simulink model "Fans_trq"  (R2016b)
settings: configuration reference "CodeGenConfigSet" (kept outside this file)
values from neighbouring files (symbols this model uses):
  Fan_facTrqDemFlt2PT1_C = Calibration.Parameter    [init_Fans_trq.m]    (also in init_Fans_trq_SIL.m = Simulink.Parameter)
  Fan_facTrqDemFltPT1_C = Calibration.Parameter    [init_Fans_trq.m]    (also in init_Fans_trq_SIL.m = Simulink.Parameter)
  Fan_numFans_C = Calibration.Parameter    [init_Fans_trq.m]    (also in init_Fans_trq_SIL.m = Simulink.Parameter)
  Fan_trqDem2_CUR = Calibration.Parameter    [init_Fans_trq.m]    (also in init_Fans_trq_SIL.m = Simulink.Parameter)
  Fan_trqDem2_CURX = Calibration.Parameter    [init_Fans_trq.m]    (also in init_Fans_trq_SIL.m = Simulink.Parameter)
  Fan_trqDem_CUR = Calibration.Parameter    [init_Fans_trq.m]    (also in init_Fans_trq_SIL.m = Simulink.Parameter)
  Fan_trqDem_CURX = Calibration.Parameter    [init_Fans_trq.m]    (also in init_Fans_trq_SIL.m = Simulink.Parameter)
  Fan_trqSplyDem2_C = Calibration.Parameter    [init_Fans_trq.m]    (also in init_Fans_trq_SIL.m = Simulink.Parameter)
  Fan_trqSplyDem_C = Calibration.Parameter    [init_Fans_trq.m]    (also in init_Fans_trq_SIL.m = Simulink.Parameter)
undefined symbols (not defined in the file or in its folder): FanCtl_facCorSpd_MAP_CURX
libraries: CXLib x4
settings Model: Creator=xinchangran  LastModifiedBy=xinchangran
settings ConfigSetRef: SourceLocation=Base Workspace

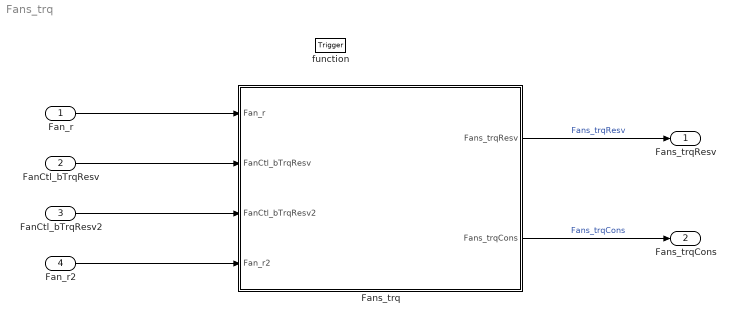
== system Fans_trq ==
  Fan_r : Inport  Tag=%  Description=Actuator setpoint value for the first fan output  OutMin=0  OutMax=100  OutDataTypeStr=DutyCycle_rate
  FanCtl_bTrqResv : Inport  Description=the additional torque required for Fan1 from the engine  Port=2  OutMin=0  OutMax=1  OutDataTypeStr=boolean
  FanCtl_bTrqResv2 : Inport  Description=the additional torque required for Fan2 from the engine  Port=3  OutMin=0  OutMax=1  OutDataTypeStr=boolean
  Fan_r2 : Inport  Tag=%  Description=set point duty cycle for PWM fan power stage 2  Port=4  OutMin=0  OutMax=100  OutDataTypeStr=DutyCycle_rate
  function : TriggerPort  TriggerType=function-call  VariantControl=Variant
  Fans_trq : Subsystem
  Fans_trqResv : Outport  Tag=Nm  Description=Torque reserve for cooling fan  OutMin=-3000  OutMax=3000  OutDataTypeStr=Trq_Nm
  Fans_trqCons : Outport  Tag=Nm  Description=Torque consumed by Fan  Port=2  OutMin=-3000  OutMax=3000  OutDataTypeStr=Trq_Nm
  wires:
  Fan_r/1 -> Fans_trq/1(Fan_r)
  FanCtl_bTrqResv/1 -> Fans_trq/2(FanCtl_bTrqResv)
  FanCtl_bTrqResv2/1 -> Fans_trq/3(FanCtl_bTrqResv2)
  Fan_r2/1 -> Fans_trq/4(Fan_r2)
  Fans_trq/1(Fans_trqResv) -> Fans_trqResv/1  "Fans_trqResv"
  Fans_trq/2(Fans_trqCons) -> Fans_trqCons/1  "Fans_trqCons"

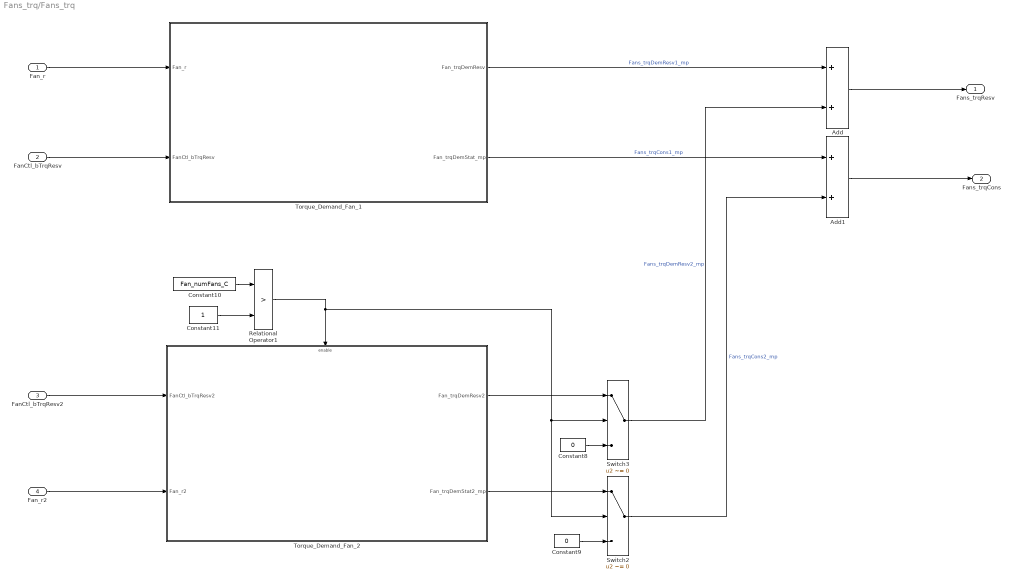
== system Fans_trq/Fans_trq ==
  Fan_r : Inport  Tag=%
  FanCtl_bTrqResv : Inport  Description=the additional torque required for Fan1 from the engine  Port=2
  FanCtl_bTrqResv2 : Inport  Description=the additional torque required for Fan2 from the engine  Port=3
  Fan_r2 : Inport  Tag=%  Port=4
  Add : Sum  SaturateOnIntegerOverflow=on  InputSameDT=on
  Add1 : Sum  SaturateOnIntegerOverflow=on  InputSameDT=on
  Constant10 : Constant  Value=Fan_numFans_C
  Constant11 : Constant  OutDataTypeStr=Inherit: Inherit via back propagation
  Constant8 : Constant  Value=0  OutDataTypeStr=Inherit: Inherit via back propagation
  Constant9 : Constant  Value=0  OutDataTypeStr=Inherit: Inherit via back propagation
  Relational Operator1 : RelationalOperator  Operator=>  OutDataTypeStr=boolean  RndMeth=Simplest
  Switch2 : Switch  Criteria=u2 ~= 0  SaturateOnIntegerOverflow=on  InputSameDT=on
  Switch3 : Switch  Criteria=u2 ~= 0  SaturateOnIntegerOverflow=on  InputSameDT=on
  Torque_Demand_Fan_1 : Subsystem
  Torque_Demand_Fan_2 : Subsystem
  Fans_trqResv : Outport
  Fans_trqCons : Outport  Port=2
  wires:
  Constant10/1 -> Relational Operator1/1
  Add/1 -> Fans_trqResv/1
  Switch2/1 -> Add1/2  "Fans_trqCons2_mp"
  Constant11/1 -> Relational Operator1/2
  Fan_r/1 -> Torque_Demand_Fan_1/1(Fan_r)
  FanCtl_bTrqResv/1 -> Torque_Demand_Fan_1/2(FanCtl_bTrqResv)
  FanCtl_bTrqResv2/1 -> Torque_Demand_Fan_2/1(FanCtl_bTrqResv2)
  Fan_r2/1 -> Torque_Demand_Fan_2/2(Fan_r2)
  Add1/1 -> Fans_trqCons/1
  Relational Operator1/1 -> Switch2/2, Switch3/2, Torque_Demand_Fan_2/Enable
  Constant8/1 -> Switch3/3
  Constant9/1 -> Switch2/3
  Torque_Demand_Fan_2/2(Fan_trqDemStat2_mp) -> Switch2/1
  Torque_Demand_Fan_1/1(Fan_trqDemResv) -> Add/1  "Fans_trqDemResv1_mp"
  Torque_Demand_Fan_2/1(Fan_trqDemResv2) -> Switch3/1
  Switch3/1 -> Add/2  "Fans_trqDemResv2_mp"
  Torque_Demand_Fan_1/2(Fan_trqDemStat_mp) -> Add1/1  "Fans_trqCons1_mp"

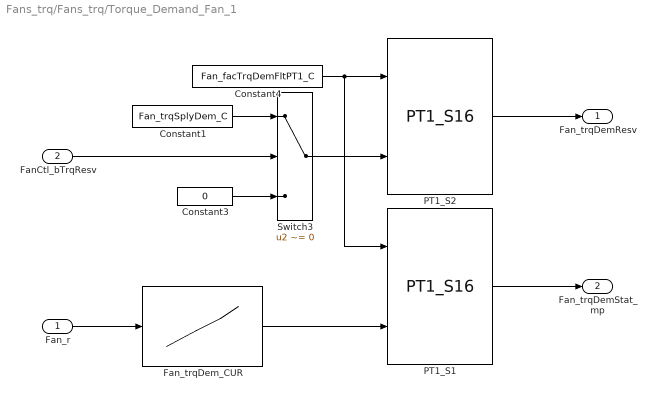
== system Fans_trq/Fans_trq/Torque_Demand_Fan_1 ==
  Fan_r : Inport  Tag=%
  FanCtl_bTrqResv : Inport  Tag=%  Port=2
  Constant1 : Constant  Value=Fan_trqSplyDem_C
  Constant3 : Constant  Value=0  OutDataTypeStr=Inherit: Inherit via back propagation
  Constant4 : Constant  Value=Fan_facTrqDemFltPT1_C
  Fan_trqDem_CUR : Lookup_n-D  NumberOfTableDimensions=1  BreakpointsForDimension1=Fan_trqDem_CURX  BreakpointsForDimension2=FanCtl_facCorSpd_MAP_CURX  IndexSearchMethod=Linear search  BeginIndexSearchUsingPreviousIndexResult=on  Table=Fan_trqDem_CUR  ExtrapMethod=Clip  UseLastTableValue=on  InternalRulePriority=Speed  OutDataTypeStr=Inherit: Inherit via back propagation  SaturateOnIntegerOverflow=on
  PT1_S1 : CXLib/PT1_S16
  PT1_S2 : CXLib/PT1_S16
  Switch3 : Switch  Criteria=u2 ~= 0  SaturateOnIntegerOverflow=on  InputSameDT=on
  Fan_trqDemResv : Outport
  Fan_trqDemStat_mp : Outport  Port=2  OutDataTypeStr=Trq_Nm
  wires:
  Fan_r/1 -> Fan_trqDem_CUR/1
  Fan_trqDem_CUR/1 -> PT1_S1/2
  PT1_S1/1 -> Fan_trqDemStat_mp/1
  Constant4/1 -> PT1_S1/1, PT1_S2/1
  FanCtl_bTrqResv/1 -> Switch3/2
  Constant1/1 -> Switch3/1
  Constant3/1 -> Switch3/3
  Switch3/1 -> PT1_S2/2
  PT1_S2/1 -> Fan_trqDemResv/1

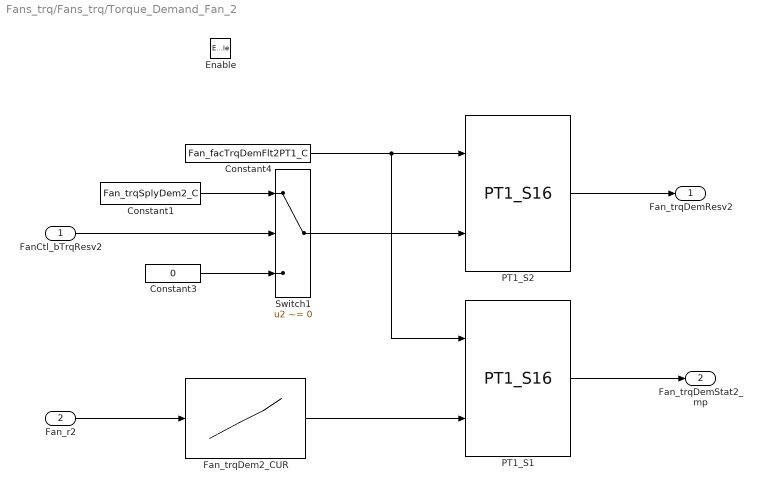
== system Fans_trq/Fans_trq/Torque_Demand_Fan_2 ==
  FanCtl_bTrqResv2 : Inport  Tag=%
  Fan_r2 : Inport  Tag=%  Port=2  OutDataTypeStr=DutyCycle_rate
  Enable : EnablePort
  Constant1 : Constant  Value=Fan_trqSplyDem2_C
  Constant3 : Constant  Value=0  OutDataTypeStr=Inherit: Inherit via back propagation
  Constant4 : Constant  Value=Fan_facTrqDemFlt2PT1_C
  Fan_trqDem2_CUR : Lookup_n-D  NumberOfTableDimensions=1  BreakpointsForDimension1=Fan_trqDem2_CURX  BreakpointsForDimension2=FanCtl_facCorSpd_MAP_CURX  IndexSearchMethod=Linear search  BeginIndexSearchUsingPreviousIndexResult=on  Table=Fan_trqDem2_CUR  ExtrapMethod=Clip  UseLastTableValue=on  InternalRulePriority=Speed  OutDataTypeStr=Inherit: Inherit via back propagation  SaturateOnIntegerOverflow=on
  PT1_S1 : CXLib/PT1_S16
  PT1_S2 : CXLib/PT1_S16
  Switch1 : Switch  Criteria=u2 ~= 0  SaturateOnIntegerOverflow=on  InputSameDT=on
  Fan_trqDemResv2 : Outport
  Fan_trqDemStat2_mp : Outport  Port=2  OutDataTypeStr=Trq_Nm
  wires:
  Fan_r2/1 -> Fan_trqDem2_CUR/1
  Fan_trqDem2_CUR/1 -> PT1_S1/2
  Constant4/1 -> PT1_S1/1, PT1_S2/1
  FanCtl_bTrqResv2/1 -> Switch1/2
  Constant1/1 -> Switch1/1
  Constant3/1 -> Switch1/3
  Switch1/1 -> PT1_S2/2
  PT1_S2/1 -> Fan_trqDemResv2/1
  PT1_S1/1 -> Fan_trqDemStat2_mp/1
